simulink model "BiglideModel"  (R2020a)
settings: Solver=VariableStepAuto  StartTime=0.0  StopTime=5  RelTol=1e-3
values from neighbouring files (symbols this model uses):
  ADAMS_communication_interval = 0.005    [ControlsPlantModel.m]
  ADAMS_communications_per_output_step = 1    [ControlsPlantModel.m]
  ADAMS_cwd = 'C:\Users\Gowri Umesh\OneDrive\Desktop\RAJEEV_UMESH_AMORO_Report\ModelVerification'    [ControlsPlantModel.m]
  ADAMS_exec = ''    [ControlsPlantModel.m]
  ADAMS_host = 'DESKTOP-1FI5JCT'    [ControlsPlantModel.m]
  ADAMS_init = ''    [ControlsPlantModel.m]
  ADAMS_inputs = 'q1!q2'    [ControlsPlantModel.m]
  ADAMS_outputs = 'x!y!xd!yd!xdd!ydd!phi1!phi2!phi1d!phi2d!phi1dd!phi2dd!f1!f2'    [ControlsPlantModel.m]
  ADAMS_prefix = 'ControlsPlantModel'    [ControlsPlantModel.m]
  ADAMS_static = 'no'    [ControlsPlantModel.m]
  ADAMS_sysdir = 'C:\PROGRA~1\MSC~1.SOF\ADAMSS~1\2020_1\'    [ControlsPlantModel.m]
  ADAMS_time_offset = 0.0    (= 0)    [ControlsPlantModel.m]
settings Model: Creator=Gowri Umesh  LastModifiedBy=Gowri Umesh

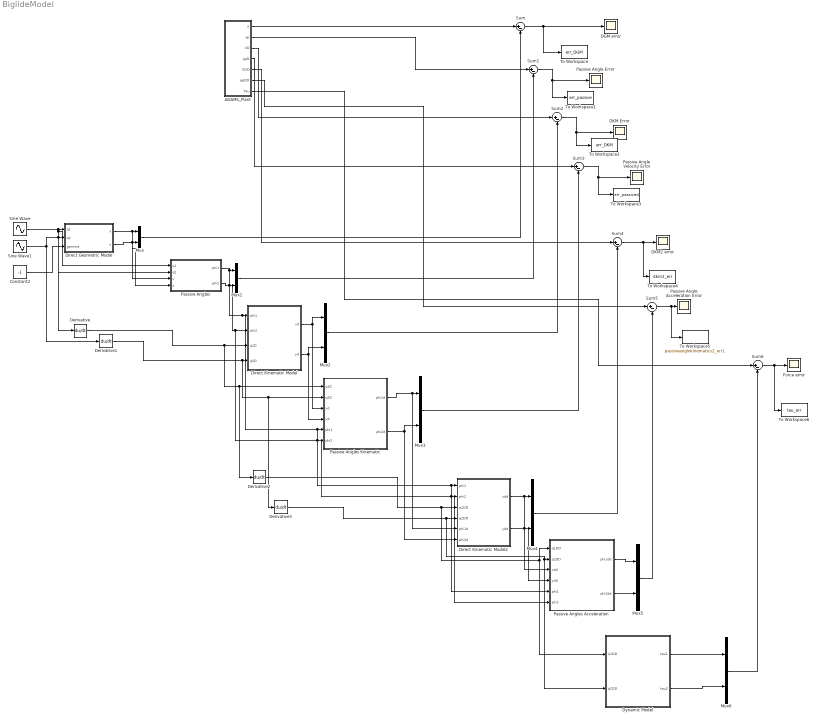
== system BiglideModel ==
  ADAMS_Plant : Subsystem
  Constant2 : Constant  Value=-1
  DGM error : Scope
  DKM Error : Scope
  DKM2 error : Scope
  Derivative{,1..3} (4 alike) : Derivative
  Direct Geometric Model : MATLAB Function  TreatAsAtomicUnit=on
  Direct Kinematic Model : MATLAB Function  TreatAsAtomicUnit=on
  Direct Kinematic Model2 : MATLAB Function  TreatAsAtomicUnit=on
  Dynamic Model : MATLAB Function  TreatAsAtomicUnit=on
  Force error : Scope
  Mux{,1..6} (7 alike) : Mux  Inputs=2
  Passive Angle Acceleration Error : Scope
  Passive Angle Error : Scope
  Passive Angle Velocity Error : Scope
  Passive Angles : MATLAB Function  TreatAsAtomicUnit=on
  "Passive Angles Acceleration " : MATLAB Function  TreatAsAtomicUnit=on
  Passive Angles Kinematic : MATLAB Function  TreatAsAtomicUnit=on
  Sine Wave : Sin  Amplitude=0.1  SampleTime=0
  Sine Wave1 : Sin  Amplitude=-0.1  SampleTime=0
  Sum{,1..6} (7 alike) : Sum  Inputs=|+-
  To Workspace : ToWorkspace  VariableName=err_DGM  SaveFormat=Timeseries  SampleTime=-1
  To Workspace1 : ToWorkspace  VariableName=err_passive  SaveFormat=Timeseries  SampleTime=-1
  To Workspace2 : ToWorkspace  VariableName=err_DKM  SaveFormat=Timeseries  SampleTime=-1
  To Workspace3 : ToWorkspace  VariableName=err_passived  SaveFormat=Timeseries  SampleTime=-1
  To Workspace4 : ToWorkspace  VariableName=dkm2_err  SaveFormat=Timeseries  SampleTime=-1
  To Workspace5 : ToWorkspace  VariableName=passiveanglekinematics2_err1  SaveFormat=Timeseries  SampleTime=-1
  To Workspace6 : ToWorkspace  VariableName=tau_err  SaveFormat=Timeseries  SampleTime=-1
  wires:
  Direct Kinematic Model/2(yd) -> Mux2/2, Passive Angles Kinematic/4(yd)
  Passive Angles/1(phi1) -> "Passive Angles Acceleration "/5(phi1), Direct Kinematic Model2/1(phi1), Passive Angles Kinematic/5(phi1), Direct Kinematic Model/1(phi1), Mux1/1
  ADAMS_Plant/2(qp) -> Sum1/1
  Sum1/1 -> Passive Angle Error/1, To Workspace1/1
  Passive Angles/2(phi2) -> "Passive Angles Acceleration "/6(phi2), Direct Kinematic Model2/2(phi2), Passive Angles Kinematic/6(phi2), Direct Kinematic Model/2(phi2), Mux1/2
  Sine Wave/1 -> Derivative/1, Passive Angles/1(q1), Direct Geometric Model/1(q1)
  ADAMS_Plant/6(qpDD) -> Sum5/1
  Direct Kinematic Model/1(xd) -> Mux2/1, Passive Angles Kinematic/3(xd)
  ADAMS_Plant/1(X) -> Sum/1
  Passive Angles Kinematic/1(phi1d) -> Direct Kinematic Model2/5(phi1d), Mux3/1
  ADAMS_Plant/5(XDD) -> Sum4/1
  Mux1/1 -> Sum1/2
  Mux3/1 -> Sum3/2
  Sine Wave1/1 -> Derivative1/1, Passive Angles/2(q2), Direct Geometric Model/2(q2)
  Mux2/1 -> Sum2/2
  Sum2/1 -> DKM Error/1, To Workspace2/1
  Direct Geometric Model/1(x) -> Passive Angles/3(x), Mux/1
  ADAMS_Plant/3(XD) -> Sum2/1
  Direct Geometric Model/2(y) -> Passive Angles/4(y), Mux/2
  Passive Angles Kinematic/2(phi2d) -> Direct Kinematic Model2/6(phi2d), Mux3/2
  Sum/1 -> DGM error/1, To Workspace/1
  Sum3/1 -> Passive Angle Velocity Error/1, To Workspace3/1
  ADAMS_Plant/4(qpD) -> Sum3/1
  Mux/1 -> Sum/2
  Derivative/1 -> Passive Angles Kinematic/1(q1D), Derivative2/1, Direct Kinematic Model/3(q1D)
  Derivative1/1 -> Derivative3/1, Passive Angles Kinematic/2(q2D), Direct Kinematic Model/4(q2D)
  Constant2/1 -> Direct Geometric Model/3(gamma)
  Derivative2/1 -> Direct Kinematic Model2/3(q1DD), Dynamic Model/1(q1DD), "Passive Angles Acceleration "/1(q1DD)
  Derivative3/1 -> Direct Kinematic Model2/4(q2DD), Dynamic Model/2(q2DD), "Passive Angles Acceleration "/2(q2DD)
  Direct Kinematic Model2/1(xdd) -> "Passive Angles Acceleration "/3(xdd), Mux4/1
  Direct Kinematic Model2/2(ydd) -> "Passive Angles Acceleration "/4(ydd), Mux4/2
  Mux4/1 -> Sum4/2
  Sum4/1 -> To Workspace4/1, DKM2 error/1
  "Passive Angles Acceleration "/1(phi1dd) -> Mux5/1
  "Passive Angles Acceleration "/2(phi2dd) -> Mux5/2
  Mux5/1 -> Sum5/2
  Sum5/1 -> To Workspace5/1, Passive Angle Acceleration Error/1
  Dynamic Model/1(tau1) -> Mux6/1
  Dynamic Model/2(tau2) -> Mux6/2
  Mux6/1 -> Sum6/2
  ADAMS_Plant/7(Tau) -> Sum6/1
  Sum6/1 -> To Workspace6/1, Force error/1

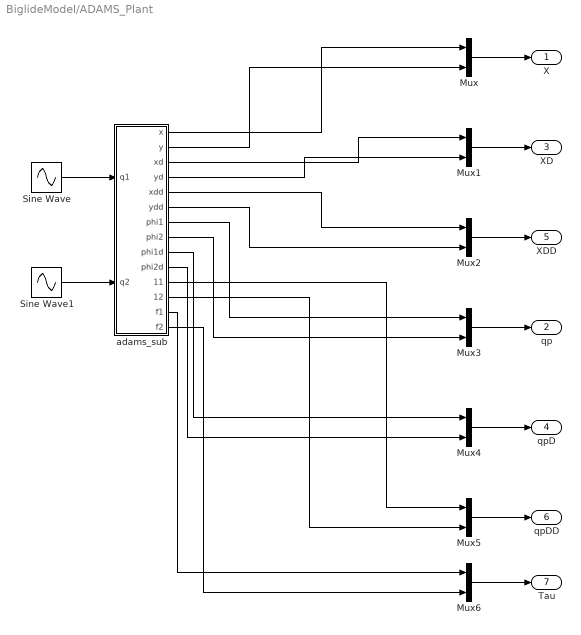
== system BiglideModel/ADAMS_Plant ==
  Mux{,1..6} (7 alike) : Mux  Inputs=2
  Sine Wave : Sin  Amplitude=0.1  SampleTime=0
  Sine Wave1 : Sin  Amplitude=-0.1  SampleTime=0
  adams_sub : Subsystem
  X : Outport
  qp : Outport  Port=2
  XD : Outport  Port=3
  qpD : Outport  Port=4
  XDD : Outport  Port=5
  qpDD : Outport  Port=6
  Tau : Outport  Port=7
  wires:
  Mux1/1 -> XD/1
  Mux/1 -> X/1
  Mux2/1 -> XDD/1
  Mux5/1 -> qpDD/1
  Mux4/1 -> qpD/1
  Mux3/1 -> qp/1
  Sine Wave/1 -> adams_sub/1(q1)
  Sine Wave1/1 -> adams_sub/2(q2)
  adams_sub/1("x     ") -> Mux/1
  adams_sub/2("y     ") -> Mux/2
  adams_sub/3("xd    ") -> Mux1/1
  adams_sub/4("yd    ") -> Mux1/2
  adams_sub/5("xdd   ") -> Mux2/1
  adams_sub/6("ydd   ") -> Mux2/2
  adams_sub/7("phi1  ") -> Mux3/1
  adams_sub/8("phi2  ") -> Mux3/2
  adams_sub/9("phi1d ") -> Mux4/1
  adams_sub/10("phi2d ") -> Mux4/2
  adams_sub/11(phi1dd) -> Mux5/1
  adams_sub/12(phi2dd) -> Mux5/2
  Mux6/1 -> Tau/1
  adams_sub/13("f1    ") -> Mux6/1
  adams_sub/14("f2    ") -> Mux6/2

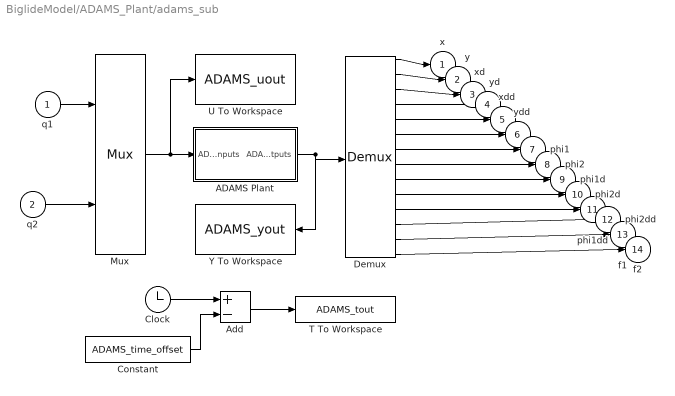
== system BiglideModel/ADAMS_Plant/adams_sub ==
  q1 : Inport
  q2 : Inport  Port=2
  ADAMS Plant : Subsystem  LoadFcn=|  InitFcn=clear mex  mask(Adams Plant){exevie=ADAMS_sysdir, nam_in=ADAMS_inputs, namout=ADAMS_outputs, nampre=ADAMS_prefix, outfil=ADAMS_prefix, exesol=ADAMS_exec, stat=ADAMS_static, inicmd=[ADAMS_init], exetyp=C++, comtyp=PIPE(DDE), workdir=ADAMS_cwd, ada_host=ADAMS_host, modani=batch, modsim=discrete, dft=no, simulink_lead_cosim=yes, pin_interp_order=0, pout_extrap_order=0, pin_extrap_order=0, pout_interp_order=0, dt_out=ADAMS_communication_interval, o_rate=ADAMS_communications_per_output_step, time_offset=ADAMS_time_offset, more=off}
      | %check based on dialog box setting for when setting by popup menu                                             
      | if exist('ADAMS_solver_type')                                                                                 
      |   if strcmp(ADAMS_solver_type,'C++')                                                                          
      |     set_param(gcb,'exetyp','C++');                                                                            
      |   else                                                                                                        
      |     set_param(gcb,'exetyp','Fortran');                                                                        
      |   end                                                                                                         
      | else                                                                                                          
      |   set_param(gcb,'exetyp','C++');                                                                              
      | end                                                                                                           
      | %set the mode if using acar_solver                                                                            
      | %REQUIRED HERE BECAUSE BELOW CAUSES MDLTERMINATE TO BE CALLED 2 TIMES IN MIDDLE OF SIMULATION WHEN SET IN MASK
      |                                                                                                               
      | %enable the direct feedthrough, sim mode, anim mode parameters by default                                     
      |                                                                                                               
      | if exist('set_some_params_states')                                                                            
      |                                                                                                               
      |   set_some_params_states({'dft','modsim','modani'},{'on','on','on'},'MaskEnables',gcb)                        
      |   %turn on direct feedthrough option                                                                          
      |   set_some_params_states({'dft'},{'on'},'MaskVisibilities',gcb)                                               
      |                                                                                                               
      |  end                                                                                                          
      |                                                                                                               
      |                                                                                                               
      | if exist('ADAMS_exec')                                                                                        
      |   if and(strcmp(get_param(gcb,'exesol'),'ADAMS_exec'),strcmp(ADAMS_exec,'acar_solver'))                       
      |     %set the sim mode to discrete -- only supported mode                                                      
      |     set_param(gcb,'modsim','discrete')                                                                        
      |      %turn off direct feedthrough option                                                                      
      |      set_some_params_states({'dft'},{'off'},'MaskVisibilities',gcb)                                           
      |     %set the animation mode to batch -- only supported mode                                                   
      |     set_param(gcb,'modani','batch')                                                                           
      |     %disable the direct feedthrough, sim mode, anim mode parameters                                           
      |     set_some_params_states({'modsim','modani'},{'off','off'},'MaskEnables',gcb)                               
      |   end
      |   if and(strcmp(get_param(gcb,'exesol'),'ADAMS_exec'),strcmp(ADAMS_exec,'apre_solver'))                       
      |     %set the sim mode to discrete -- only supported mode                                                      
      |     set_param(gcb,'modsim','discrete')                                                                        
      |      %turn off direct feedthrough option                                                                      
      |      set_some_params_states({'dft'},{'off'},'MaskVisibilities',gcb)                                           
      |     %set the animation mode to batch -- only supported mode                                                   
      |     set_param(gcb,'modani','batch')                                                                           
      |     %disable the direct feedthrough, sim mode, anim mode parameters                                           
      |     set_some_params_states({'modsim','modani'},{'off','off'},'MaskEnables',gcb)                               
      |   end                                                                                                  
      | end
      mask prompts: exevie "Adams install directory"; nam_in "Adams View input names"; namout "Adams View output names"; nampre "Adams model file prefix"; outfil "Output files prefix (opt.: if blank - no output)"; exesol "User executable (opt.: if blank - use standard)"; stat "Initial static simulation flag"; inicmd "Initialization commands"; exetyp "Adams Solver type"; comtyp "Interprocess option"; workdir "Adams working directory"; ada_host "Adams host"; modani "Animation mode"; modsim "Simulation mode"; dft "Direct feedthrough"; simulink_lead_cosim "Discrete Computational Order - Simulink Leads Adams"; pin_interp_order "Plant input interpolation order"; pout_extrap_order "Plant output extrapolation order"; pin_extrap_order "Plant input extrapolation order"; pout_interp_order "Plant output interpolation order"; dt_out "Communication interval"; o_rate "Number of communications per output step"; time_offset "Offset between Simulink and Adams simulation time"; more "More parameters"
      mask help: Simulate any Adams plant model either in Adams Solver form (.adm file) or in Adams View form (.cmd file)
      settings: OpenFcn=|
      | open_system(gcb,'mask')
      | if not(exist('set_some_params_states'))
      | 
      | warning('The script "set_some_params_states.m" cannot be found in the MATLAB PATH.  Cannot update the ADAMS Plant S-Function parameters.')
      | 
      | warning('Recommended action(optional):  run the Adams Controls .m file first to help choose the correct settings in the Adams S-Function block.')
      | 
      | end
      mask Help:
      | <html>
      | This S-Function represents the non-linear Adams Plant with the inputs sent to the Adams model as input #1 and Time as input #2<br>
      |  and the outputs generated by the Adams model.  See the Adams Controls documentation for more <br>
      | information.  This plant uses the following variables:<br>
      | <br>
      | <b>ADAMS_sysdir:</b> Adams installation directory<br>
      | <b>ADAMS_inputs:</b> Input variables View names vector<br>
      | <b>ADAMS_outputs :</b> Outputs variables View names vector<br>
      | <b>ADAMS_prefix:</b> ADAMS model files prefix (.adm, .cmd); also doubles as output files prefix<br>
      | <b>ADAMS_exec:</b>  Adams Solver user library or keyword (e.g., acar_solver)<br>
      | <b>ADAMS_static:</b> yes|no - initial static before Co-simulation(discrete)/Function Evaluation(continuous)<br>
      | <b>ADAMS_init:</b> Initialization commands (i.e., Adams View or Solver commands, depending on setting for Animation mode)<br>
      | <b>ADAMS_cwd:</b> Current working directory (for TCP/IP)<br>
      | <b>ADAMS_host:</b> Name of Adams server host (for TCP/IP)<br>
      | <b>ADAMS_mode:</b> Linear or non-linear (i.e., co-sim, function eval)<br>
      | <b>ADAMS_solver_type:</b> Fortran or C++ (used to set popup menu when first loaded)<br>
      | <b>ADAMS_communication_interval:</b> Time step at which Co-simulation exchange information (e.g.,0.005); also controls <br>output for continuous mode (Function Evaluation)<br>
      | <b>ADAMS_communications_per_output_step: </b>Sets Adams output rate (.res, .req, .gra) integer value (default: 1)<br>
      | <b>ADAMS_time_offset: </b>Removes this time offset from simulation time used by Adams. Adams will be sent a time value being Simulink simulation time - this value. (default: 0). Eg. if ADAMS_time_offset=2: if Simulink time=2 then Adams time = 0. Make sure that the Adams block is disabled when the Adams time is <0. If not an error will be raised. <br>
      | 
      | 
      | <br>
      | The following settings can be chosen:<br>
      | <br>
      | <b>Adams Solver type:</b>  Fortran or C++ (will also set ADAMS_solver_type)<br>
      | <b>Interprocess option:</b> Pipe(DDE), TCP/IP or DIRECT; TCP/IP can allow different machines run Adams and MATLAB<br>
      | <b>Animation mode:</b> batch (Solver, uses .adm) or interactive (View, uses .cmd)<br>
      | <b>Simulation mode:</b> discrete (Co-simulation) or continuous (Function Evaluation)<br>
      | <b>Discrete Computational Order - Simulink Lead Adams:</b> for discrete mode, chooses if Simulink leads the integration (yes) or lags (no);<br> if set to "no", can remove algebraic loop<br>
      | <b>Plant input interpolation order:</b> 0 = zero-order hold; 1 = linear (discrete mode only, where Simulink leads)<br>
      | <b>Plant output extrapolation order:</b> 0 = zero-order hold;1 = linear(discrete mode only, where Simulink leads)<br>
      | <b>Plant input extrapolation order:</b> 0 = zero-order hold; 1 = linear (discrete mode only, where Adams leads)<br>
      | <b>Plant output interpolation order:</b> 0 = zero-order hold;1 = linear(discrete mode only, where Adams leads)<br>
      | <b>Direct feedthrough:</b> yes|no - yes = Input directly effect output(continuous mode-only)<br>
      | 
      | </html>
      mask Callback exesol:
      | if exist('set_some_params_states')
      | %enable the direct feedthrough, sim mode, anim mode parameters
      | set_some_params_states({'dft','modsim','modani'},{'on','on','on'},'MaskEnables',gcb)
      | %turn on direct feedthrough option
      | set_some_params_states({'dft'},{'on'},'MaskVisibilities',gcb)
      | end
      | 
      | if exist('ADAMS_exec')
      |   if and(strcmp(get_param(gcb,'exesol'),'ADAMS_exec'),strcmp(ADAMS_exec,'acar_solver'))
      |     %set the sim mode to discrete -- only supported mode
      |     %REMOVED:  BELOW CAUSES MDLTERMINATE TO BE CALLED 2 TIMES IN MIDDLE OF SIMULATION
      |     %Now in LoadFcn callback
      |     %set_param(gcb,'modsim','discrete')
      |      %turn off direct feedthrough option
      |     set_some_params_states({'dft'},{'off'},'MaskVisibilities',gcb)
      |     %set the animation mode to batch -- only supported mode
      |     %REMOVED:  BELOW CAUSES MDLTERMINATE TO BE CALLED 2 TIMES IN MIDDLE OF SIMULATION
      |     %Now in LoadFcn callback
      |     %set_param(gcb,'modani','batch')
      |     %disable the direct feedthrough, sim mode, anim mode parameters
      |     set_some_params_states({'modsim','modani'},{'off','off'},'MaskEnables',gcb)
      |   end
      | end
      mask TypeOptions exetyp: Fortran | C++
      mask Callback exetyp:
      | if strcmp(get_param(gcb,'exetyp'),'C++')
      |     ADAMS_solver_type='C++';
      | else
      |     ADAMS_solver_type='Fortran';
      | end
      mask TypeOptions comtyp: PIPE(DDE) | TCP/IP | DIRECT
      mask Callback comtyp:
      | if exist('set_some_params_states')
      | if strcmp(get_param(gcb,'comtyp'),'PIPE(DDE)') || strcmp(get_param(gcb,'comtyp'),'DIRECT')
      |     %turn off cwd, host options
      |     set_some_params_states({'ada_host','workdir'},{'off','off'},'MaskVisibilities',gcb)
      | else%if strcmp(get_param(gcb,'modsim'),'TCP/IP')
      |     %turn on cwd, host options
      |     set_some_params_states({'ada_host','workdir'},{'on','on'},'MaskVisibilities',gcb)
      | end
      | end
      mask TypeOptions modani: batch | interactive
      mask TypeOptions modsim: discrete | continuous
      mask Callback modsim:
      | if exist('set_some_params_states')
      | if strcmp(get_param(gcb,'modsim'),'discrete')
      |      %turn off direct feedthrough option
      |     set_some_params_states({'dft'},{'off'},'MaskVisibilities',gcb)
      |     %turn on discrete co-sim type if want to see more
      |     if strcmp(get_param(gcb,'more'),'on')
      |         set_some_params_states({'simulink_lead_cosim'},{'on'},'MaskVisibilities',gcb)
      |     end
      |     if strcmp(get_param(gcb,'simulink_lead_cosim'),'yes')
      |         %turn on interpolation/extrapolation options
      |         set_some_params_states({'pin_interp_order','pout_extrap_order',},{'on','on'},'MaskVisibilities',gcb)
      |     else
      |         set_some_params_states({'pin_extrap_order','pout_interp_order'},{'on','on'},'MaskVisibilities',gcb)
      |     end
      | else%if strcmp(get_param(gcb,'modsim'),'continuous')
      |      %turn off direct feedthrough option
      |     set_some_params_states({'dft'},{'on'},'MaskVisibilities',gcb)
      |     %turn off interpolation/extrapolation options
      |     set_some_params_states({'pin_interp_order','pout_extrap_order','pin_extrap_order','pout_interp_order','simulink_lead_cosim'},{'off','off','off','off','off'},'MaskVisibilities',gcb)
      | end
      | end
      mask TypeOptions dft: no | yes
      mask TypeOptions simulink_lead_cosim: yes | no
      mask Callback simulink_lead_cosim:
      | if exist('set_some_params_states')
      | if (strcmp(get_param(gcb,'simulink_lead_cosim'),'yes') && strcmp(get_param(gcb,'modsim'),'discrete'))
      |      %turn off unused interpolate/extrapolate options
      |     set_some_params_states({'pin_extrap_order','pout_interp_order'},{'off','off'},'MaskVisibilities',gcb)
      |     %turn on used interpolate/extrapolate options
      |     set_some_params_states({'pin_interp_order','pout_extrap_order'},{'on','on'},'MaskVisibilities',gcb)
      | elseif (strcmp(get_param(gcb,'simulink_lead_cosim'),'no') && strcmp(get_param(gcb,'modsim'),'discrete'))
      |     %turn on used interpolate/extrapolate options
      |     set_some_params_states({'pin_extrap_order','pout_interp_order'},{'on','on'},'MaskVisibilities',gcb)
      |      %turn off unused interpolate/extrapolate options
      |     set_some_params_states({'pin_interp_order','pout_extrap_order'},{'off','off'},'MaskVisibilities',gcb)
      | end
      | end
      mask TypeOptions pin_interp_order: 0 | 1
      mask TypeOptions pout_extrap_order: 0 | 1
      mask TypeOptions pin_extrap_order: 0 | 1
      mask TypeOptions pout_interp_order: 0 | 1
      mask Callback more:
      | if exist('set_some_params_states')
      | if (strcmp(get_param(gcb,'more'),'on'))
      |      %turn on infrequently used options
      |     set_some_params_states({'exevie','nam_in','namout','exesol','stat','inicmd','time_offset'},{'on','on','on','on','on','on','on'},'MaskVisibilities',gcb)
      |     if strcmp(get_param(gcb,'modsim'),'discrete')
      |         set_some_params_states({'simulink_lead_cosim'},{'on'},'MaskVisibilities',gcb)
      |     end
      | elseif (strcmp(get_param(gcb,'more'),'off'))
      |     %turn off infrequently used options
      |     set_some_params_states({'exevie','nam_in','namout','exesol','stat','inicmd','time_offset'},{'off','off','off','off','off','off','off'},'MaskVisibilities',gcb)
      |     if strcmp(get_param(gcb,'modsim'),'discrete')
      |         set_some_params_states({'simulink_lead_cosim'},{'off'},'MaskVisibilities',gcb)
      |     end
      | end
      | end
      mask Display: disp( 'MSC Software' )
  Add : Sum  Inputs=+-
  Clock : Clock
  Constant : Constant  Value=ADAMS_time_offset
  Demux : Demux  Outputs=14
      settings: DisplayOption=none
  Mux : Mux  Inputs=2
  T To Workspace : ToWorkspace  VariableName=ADAMS_tout
      settings: MaxDataPoints=100000
  U To Workspace : ToWorkspace  VariableName=ADAMS_uout
      settings: MaxDataPoints=100000
  Y To Workspace : ToWorkspace  VariableName=ADAMS_yout
      settings: MaxDataPoints=100000
  "x     " : Outport
  "y     " : Outport  Port=2
  "xd    " : Outport  Port=3
  "yd    " : Outport  Port=4
  "xdd   " : Outport  Port=5
  "ydd   " : Outport  Port=6
  "phi1  " : Outport  Port=7
  "phi2  " : Outport  Port=8
  "phi1d " : Outport  Port=9
  "phi2d " : Outport  Port=10
  phi1dd : Outport  Port=11
  phi2dd : Outport  Port=12
  "f1    " : Outport  Port=13
  "f2    " : Outport  Port=14
  wires:
  Mux/1 -> ADAMS Plant/1(ADAMS inputs), U To Workspace/1
  ADAMS Plant/1(ADAMS outputs) -> Demux/1, Y To Workspace/1
  Clock/1 -> Add/1
  Constant/1 -> Add/2
  Add/1 -> T To Workspace/1
  Demux/1 -> "x     "/1
  Demux/2 -> "y     "/1
  Demux/3 -> "xd    "/1
  Demux/4 -> "yd    "/1
  Demux/5 -> "xdd   "/1
  Demux/6 -> "ydd   "/1
  Demux/7 -> "phi1  "/1
  Demux/8 -> "phi2  "/1
  Demux/9 -> "phi1d "/1
  Demux/10 -> "phi2d "/1
  Demux/11 -> phi1dd/1
  Demux/12 -> phi2dd/1
  Demux/13 -> "f1    "/1
  Demux/14 -> "f2    "/1
  q1/1 -> Mux/1
  q2/1 -> Mux/2

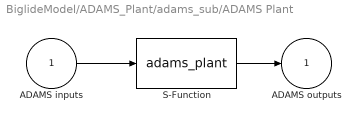
== system BiglideModel/ADAMS_Plant/adams_sub/ADAMS Plant ==
  ADAMS inputs : Inport
  S-Function : S-Function  StopFcn=clear mex  FunctionName=adams_plant  Parameters=exevie,exesol,stat,outfil,nampre,o_rate,nam_in,namout,dft,modsim,modani,dt_out,inicmd,exetyp,comtyp,ada_host, workdir,pin_interp_order,pout_extrap_order,pin_extrap_order,pout_interp_order,simulink_lead_cosim,time_offset  SFunctionDeploymentMode=off  EnableBusSupport=off
  ADAMS outputs : Outport  InitialOutput=0
  wires:
  ADAMS inputs/1 -> S-Function/1
  S-Function/1 -> ADAMS outputs/1

== matlab function BiglideModel/Passive Angles ==
  data: q1 input; phi1 output; q2 input; x input; phi2 output; y input
function [phi1,phi2] = passive_angles(q1,q2,x,y)
d = 0.4;
phi1 = atan2((y-q1),(x+(d/2)));
phi2 = atan2((y-q2),(x-(d/2)));
end

== matlab function BiglideModel/Direct Geometric Model ==
  data: q1 input; x output; q2 input; y output; gamma input
function [x,y] = DGM(q1,q2,gamma)
l = 0.3606;
d = 0.4;
E =[0 -1;1 0];

OB = [d/2;0];
OA = [-d/2;0];
AA1 = [0;q1];
BA2 = [0;q2];
OA1 = OA+AA1;

A2A1 = (-BA2-OB+AA1+OA);

A2M = 0.5*(A2A1);

a = norm(A2M);
h =sqrt(l*l - a*a);
MC = gamma*(h/a)*E*A2M;

X = OB+BA2+A2M+MC;
x = X(1);
y = X(2);
end

== matlab function BiglideModel/Direct Kinematic Model ==
  data: phi1 input; phi2 input; q1D input; q2D input; xd output; yd output
function [xd,yd] = DKM(phi1,phi2,q1D,q2D)


U1 = [cos(phi1);sin(phi1)];
U2 = [cos(phi2);sin(phi2)];

A = [transpose(U1);transpose(U2)];
B = [sin(phi1) 0;0 sin(phi2)];

pdot = inv(A)*B*[q1D;q2D];

xd = pdot(1);
yd = pdot(2);

end

== matlab function BiglideModel/Passive Angles Kinematic ==
  data: q1D input; q2D input; xd input; yd input; phi1 input; phi2 input; phi1d output; phi2d output
function [phi1d,phi2d] = passive_angleskm(q1D,q2D,xd,yd,phi1,phi2)
l = 0.3606;
E = [0 -1;1 0];
U1 = [0;1];
U2 = U1;

V1 = [cos(phi1);sin(phi1)];
V2 = [cos(phi2);sin(phi2)];
% Jtd = [l 0;0 l];
% Jt = [-sin(phi1) cos(phi1);-sin(phi2) cos(phi2)];
% Jta = [cos(phi1) 0;0 cos(phi2)];
Jtd = [l 0;0 l];
Jt = [transpose(E*V1);transpose(E*V2)];
Jta = [transpose(E*V1)*U1 0; 0 transpose(E*V2)*U2];
qD = inv(Jtd)*((Jt*[xd;yd]) -( Jta * [q1D;q2D]));
phi1d = qD(1);
phi2d = qD(2);
end

== matlab function BiglideModel/Direct Kinematic Model2 ==
  data: phi1 input; phi2 input; q1DD input; q2DD input; xdd output; ydd output; phi1d input; phi2d input
function [xdd,ydd] = DKM2(phi1,phi2,q1DD,q2DD,phi1d,phi2d)
l = 0.3606;



V1 = [cos(phi1);sin(phi1)];
V2 = [cos(phi2);sin(phi2)];

U1 = [cos(90);sin(90)];
U2 = U1;

A = [transpose(V1);transpose(V2)];
B = [transpose(V1)*U1 0;0 transpose(V2)*U2];
C = [l 0;0 l];

pddot = inv(A)*(B*[q1DD;q2DD] - C*[phi1d^2;phi2d^2]);

xdd = pddot(1);
ydd = pddot(2);

end

== matlab function BiglideModel/Passive Angles Acceleration  ==
  data: q1DD input; q2DD input; xdd input; ydd input; phi1 input; phi2 input; phi1dd output; phi2dd output
function [phi1dd,phi2dd] = passive_angleskm2(q1DD,q2DD,xdd,ydd,phi1,phi2)
l = 0.3606;
V1 = [cos(phi1);sin(phi1)];
V2 = [cos(phi2);sin(phi2)];

U1 = [cos(90);sin(90)];
U2 = U1;

E = [0 -1;1 0];
A = [l 0;0 l];
B = [transpose(E*V1);transpose(E*V2)];
C = [transpose(E*V1)*U1 0;0 transpose(E*V2)*U2];

qDD = inv(A)*((B*[xdd;ydd]) -( C * [q1DD;q2DD]));
phi1dd = qDD(1);
phi2dd = qDD(2);
end

== matlab function BiglideModel/Dynamic Model ==
  data: q1DD input; q2DD input; tau1 output; tau2 output
function [tau1,tau2] = passive_angleskm2(q1DD,q2DD)
m = 1;
tau = [m 0;0 m]*[q1DD;q2DD];
tau1 = tau(1);
tau2 = tau(2);

end
